simulink model "sensor_development"  (R2025b)
settings: Solver=VariableStepAuto  StartTime=0.0  StopTime=10.0  RelTol=1e-3
settings Model: Creator=atcushen  LastModifiedBy=atcushen

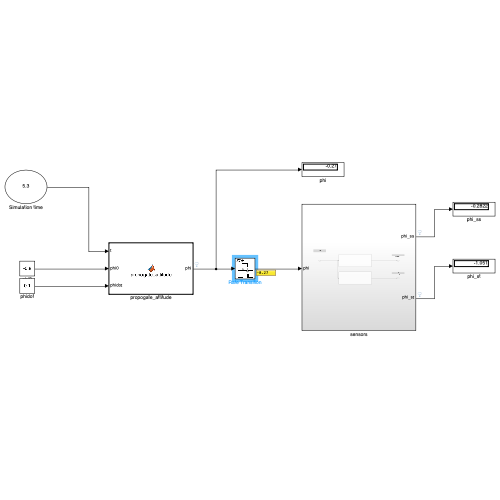
[thumbnail: Simulink's stored preview of the top-level diagram]
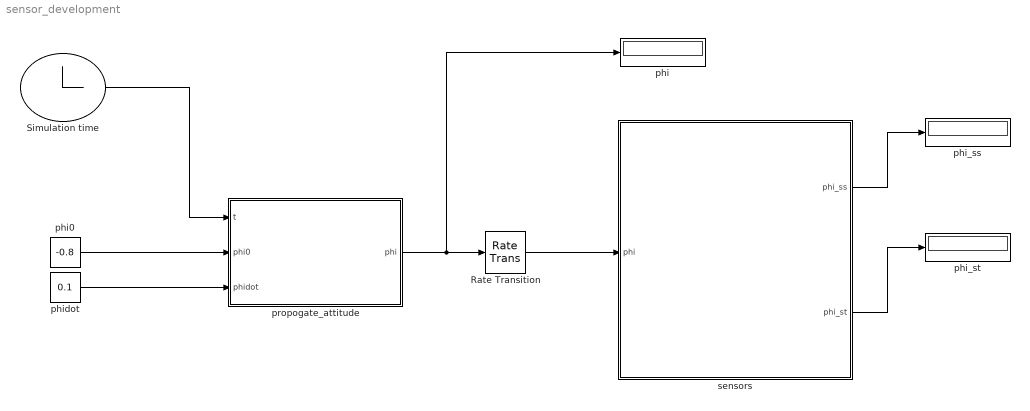
== system sensor_development ==
  Rate Transition : RateTransition  OutPortSampleTime=0.1
  Simulation time : Clock
  phi : Display
  phi0 : Constant  Value=-0.8
  phi_ss : Display
  phi_st : Display
  phidot : Constant  Value=0.1
  propogate_attitude : MATLAB Function  TreatAsAtomicUnit=on
  sensors : Subsystem
  wires:
  Simulation time/1 -> propogate_attitude/1(t)
  phi0/1 -> propogate_attitude/2(phi0)
  phidot/1 -> propogate_attitude/3(phidot)
  propogate_attitude/1(phi) -> phi/1, Rate Transition/1
  Rate Transition/1 -> sensors/1(phi)
  sensors/1(phi_ss) -> phi_ss/1
  sensors/2(phi_st) -> phi_st/1

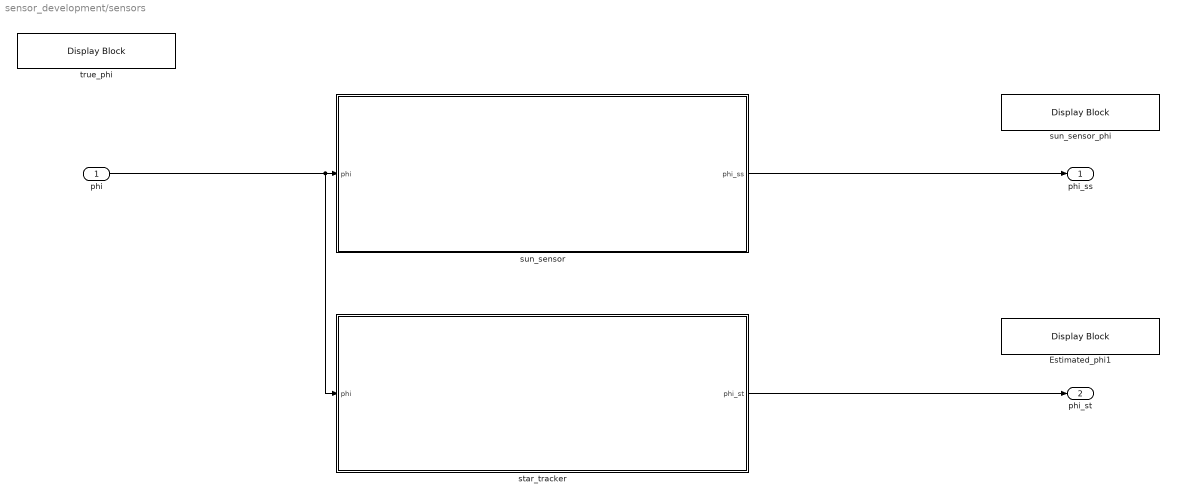
== system sensor_development/sensors ==
  phi : Inport
  Estimated_phi1 : DisplayBlock  LabelPosition=Bottom  Transparency=1  GridColor=[0.502, 0.502, 0.502]
  star_tracker : Subsystem
  sun_sensor : Subsystem
  sun_sensor_phi : DisplayBlock  LabelPosition=Bottom  Transparency=1  GridColor=[0.502, 0.502, 0.502]
  true_phi : DisplayBlock  LabelPosition=Hide  Transparency=1  GridColor=[0.502, 0.502, 0.502]
  phi_ss : Outport
  phi_st : Outport  Port=2
  wires:
  phi/1 -> star_tracker/1(phi), sun_sensor/1(phi)
  sun_sensor/1(phi_ss) -> phi_ss/1
  star_tracker/1(phi_st) -> phi_st/1

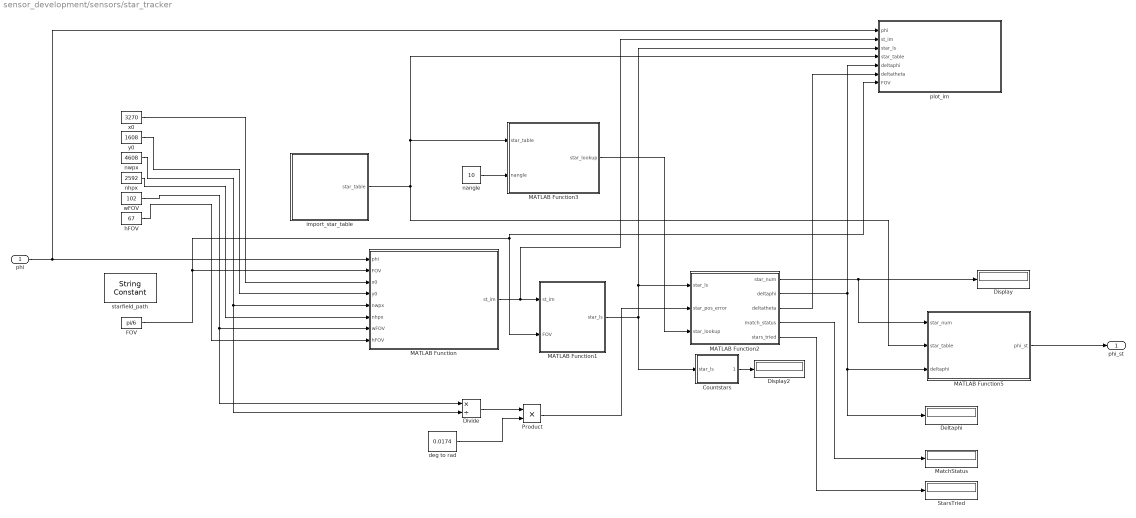
== system sensor_development/sensors/star_tracker ==
  phi : Inport
  Countstars : MATLAB Function  TreatAsAtomicUnit=on
  Deltaphi : Display
  Display : Display
  Display2 : Display
  Divide : Product  Inputs=*/
  FOV : Constant  Value=pi/6
  MATLAB Function : MATLAB Function  TreatAsAtomicUnit=on
  MATLAB Function1 : MATLAB Function  TreatAsAtomicUnit=on
  MATLAB Function2 : MATLAB Function  TreatAsAtomicUnit=on
  MATLAB Function3 : MATLAB Function  TreatAsAtomicUnit=on
  MATLAB Function5 : MATLAB Function  TreatAsAtomicUnit=on
  MatchStatus : Display
  Product : Product
  StarsTried : Display
  deg to rad : Constant  Value=0.0174
  hFOV : Constant  Value=67
  import_star_table : MATLAB Function  TreatAsAtomicUnit=on
  nangle : Constant  Value=10
  nhpx : Constant  Value=2592
  nwpx : Constant  Value=4608
  plot_im : MATLAB Function  TreatAsAtomicUnit=on
  starfield_path : StringConstant  String='star_field1.png'
  wFOV : Constant  Value=102
  x0 : Constant  Value=3270
  y0 : Constant  Value=1608
  phi_st : Outport
  wires:
  nhpx/1 -> MATLAB Function/6(nhpx)
  Countstars/1(num_stars) -> Display2/1
  nangle/1 -> MATLAB Function3/2(nangle)
  hFOV/1 -> MATLAB Function/8(hFOV)
  MATLAB Function2/4(match_status) -> MatchStatus/1
  Product/1 -> MATLAB Function2/2(star_pos_error)
  y0/1 -> MATLAB Function/4(y0)
  MATLAB Function1/1(star_ls) -> Countstars/1(star_ls), plot_im/3(star_ls), MATLAB Function2/1(star_ls)
  MATLAB Function/1(st_im) -> plot_im/2(st_im), MATLAB Function1/1(st_im)
  MATLAB Function3/1(star_lookup) -> MATLAB Function2/3(star_lookup)
  nwpx/1 -> Divide/2, MATLAB Function/5(nwpx)
  Divide/1 -> Product/1
  MATLAB Function2/5(stars_tried) -> StarsTried/1
  x0/1 -> MATLAB Function/3(x0)
  phi/1 -> plot_im/1(phi), MATLAB Function/1(phi)
  MATLAB Function2/2(deltaphi) -> Deltaphi/1, MATLAB Function5/3(deltaphi), plot_im/5(deltaphi)
  wFOV/1 -> Divide/1, MATLAB Function/7(wFOV)
  deg to rad/1 -> Product/2
  MATLAB Function2/1(star_num) -> MATLAB Function5/1(star_num), Display/1
  import_star_table/1(star_table) -> plot_im/4(star_table), MATLAB Function3/1(star_table), MATLAB Function5/2(star_table)
  FOV/1 -> MATLAB Function/2(FOV), MATLAB Function1/2(FOV), plot_im/7(FOV)
  MATLAB Function5/1(phi_st) -> phi_st/1
  MATLAB Function2/3(deltatheta) -> plot_im/6(deltatheta)

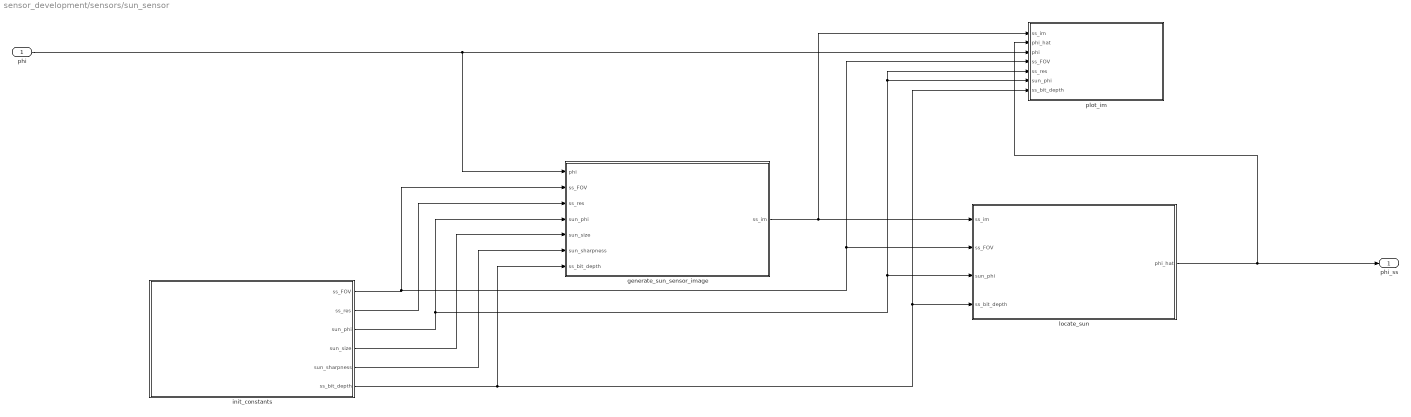
== system sensor_development/sensors/sun_sensor ==
  phi : Inport
  generate_sun_sensor_image : MATLAB Function  TreatAsAtomicUnit=on
  init_constants : MATLAB Function  TreatAsAtomicUnit=on
  locate_sun : MATLAB Function  TreatAsAtomicUnit=on
  plot_im : MATLAB Function  TreatAsAtomicUnit=on
  phi_ss : Outport
  wires:
  phi/1 -> generate_sun_sensor_image/1(phi), plot_im/3(phi)
  init_constants/5(sun_sharpness) -> generate_sun_sensor_image/6(sun_sharpness)
  generate_sun_sensor_image/1(ss_im) -> plot_im/1(ss_im), locate_sun/1(ss_im)
  locate_sun/1(phi_hat) -> phi_ss/1, plot_im/2(phi_hat)
  init_constants/1(ss_FOV) -> plot_im/4(ss_FOV), locate_sun/2(ss_FOV), generate_sun_sensor_image/2(ss_FOV)
  init_constants/2(ss_res) -> generate_sun_sensor_image/3(ss_res)
  init_constants/4(sun_size) -> generate_sun_sensor_image/5(sun_size)
  init_constants/3(sun_phi) -> generate_sun_sensor_image/4(sun_phi), plot_im/6(sun_phi), plot_im/5(ss_res), locate_sun/3(sun_phi)
  init_constants/6(ss_bit_depth) -> generate_sun_sensor_image/7(ss_bit_depth), plot_im/7(ss_bit_depth), locate_sun/4(ss_bit_depth)

== matlab function sensor_development/sensors/sun_sensor/plot_im ==
  data: ss_im input; phi_hat input; phi input; ss_FOV input; ss_res input; sun_phi input; ss_bit_depth input
function plot_im(ss_im,phi_hat,phi,ss_FOV,ss_res,sun_phi,ss_bit_depth)
   % Show synthetic image
    subplot(1, 2, 1);
    hold on
    imshow(ss_im, [], 'XData', linspace(-ss_FOV/2,ss_FOV/2,ss_res), 'YData', linspace(-ss_FOV/2,ss_FOV/2,ss_res));
    caxis([0 ss_bit_depth]); % Set the color axis limits for imshow
    % Add a vertical red line at (sun_phi - phi_hat)
    if ~isnan(phi_hat)
        xline(sun_phi - phi_hat, 'r', 'LineWidth', 2);
    end
    xline(sun_phi - phi, 'g', 'LineWidth', 2);
    set(gca, 'YDir', 'normal');
    title('Star Tracker Image'); % Title for the second subplot
    axis on
    xlabel('Azimuth (\delta\phi)');
    ylabel('Inclination (\delta\theta)');
    hold off
end

== matlab function sensor_development/sensors/star_tracker/MATLAB Function2 ==
  data: star_ls input; star_num output int32 size=1; star_pos_error input; star_lookup input; deltaphi output size=1; deltatheta output size=1; match_status output; stars_tried output
function [star_num,deltaphi,deltatheta,match_status,stars_tried] = match_to_lookup(star_ls,star_pos_error,star_lookup)
    % Input
    % star_ls: nx2 array, the phi and theta positions (relative to the
    % center of the image) for each star identified
    % star_pos_error: float, angular uncertainty in position of stars
    % star_lookup: nxnagle array, each row corresponds to given row in
    % star_table, columns are angular distances to closest stars

    % Output
    % star_num: integer, index number of matched star
    % deltaphi: float, offset in phi of matched star from image center, in
    % radians
    % deltatheta: float, offset in phi of matched star from image center,
    % in radians
    % CHANGED FOR CODEGEN - Initialize outputs with default values
    star_num = int32(-1);
    deltaphi = 0.0;
    deltatheta = 0.0;
    match_status = int32(0);  % debug output
    stars_tried = int32(0);   % debug output

    % Iterate through stars in image, starting closest to middle, until we
    % get a positive match
    star_match = false;
    
    % Calculate the sum of squares for each star position
    star_ls_dist = sum(star_ls.^2, 2);
    
    % Sort the star_ls based on the sum of squares
    [~, sorted_indices] = sort(star_ls_dist);
    star_ls = star_ls(sorted_indices, :);

    istar = 1;
    while star_match == false && istar <= length(star_ls)
        stars_tried = int32(istar);  % tracking progress
        
        % Compute distances to other stars
        phi_diff = star_ls(istar, 1) - star_ls(:, 1);
        theta_diff = star_ls(istar, 2) - star_ls(:, 2);
        angle_diff = sqrt(phi_diff.^2 + theta_diff.^2);

        % Sort the computed angular distances from smallest to largest
        [sorted_angles, ~] = sort(angle_diff);
        
        % Drop the first element of sorted_angles (distance to itself = 0)
        sorted_angles(1) = [];

        % Reduce sorted angles to only be as long as star_lookup is wide
        sorted_angles = sorted_angles(1:min(length(sorted_angles), size(star_lookup, 2)));

        % Create an array of stars within the positional error range
        match_indices = star_lookup(:, 1) >= (sorted_angles(1) - star_pos_error) & ...
                        star_lookup(:, 1) <= (sorted_angles(1) + star_pos_error);
        matched_stars = star_lookup(match_indices, :);

        % Check if that immediately identified the current state. 
        % If not, compare the angular distances one by one, bringing in more to
        % reduce the number of remaining options
        iangle = 2;

        while size(matched_stars,1) > 1 & iangle <= size(star_lookup,2)
            match_status = int32(2);  % indicates multiple matches being refined
            
            % We loop through the remaining matches
            for j = 1:size(match_indices, 1)
                if j ~= 0
                    % Check to see if the next closest star is within error of
                    % any of the neighbouring stars listed in the lookup table
                    % If none of the angles are close enough, then reject this
                    % match
                    if all(abs(star_lookup(j, iangle:end) - sorted_angles(iangle)) > star_pos_error)
                        match_indices(j) = 0; % Set the jth non-zero element of match_indices to zero
                    end
                end 
            end
            matched_stars = star_lookup(match_indices, :);
        
            iangle = iangle + 1;
        end
        
        % Check if we could use this star 
        if size(matched_stars,1) ~= 1
            % no match found for this star, continue
            istar = istar + 1; % Move to the next star
        else
            % CHANGED FOR CODEGEN - Force scalar by using loop instead of find
            for k = 1:length(match_indices)
                if match_indices(k) ~= 0
                    star_num = int32(k);
                    break;
                end
            end
            deltaphi = star_ls(istar,1); % Offset in phi
            deltatheta = star_ls(istar,2); % Offset in theta
            star_match = true;
            match_status = int32(1);  % successful match
        end
    end
    
    % Return error if star tracker failed 
    if star_match == false
        % CHANGED FOR CODEGEN - tracker failed
        star_num = int32(-1);
        deltaphi = 0.0;
        deltatheta = 0.0;
        match_status = int32(0);  % Failed to match
    end
    
end

== matlab function sensor_development/sensors/star_tracker/MATLAB Function5 ==
  data: star_num input; phi_st output; star_table input; deltaphi input
function phi_st = compute_boresight_phi(star_num,star_table,deltaphi)
    % Input
    % star_num: integer, index number of matched star
    % star_table: n_stars x 3 array, where column 1 is phi position of
    % star, column 2 is theta position, column 3 is relative brightness
    % deltaphi: float, offset in phi of matched star from image center, in
    % radians
    
    % Output
    % boresight_phi: float, actual orientation of the center of the cameras
    % FOV [rad]
    
    if star_num<0
        phi_st = NaN;
    else
        phi_st = star_table(star_num,1) - deltaphi;
    end
end

== matlab function sensor_development/sensors/star_tracker/Countstars ==
  data: star_ls input; num_stars output
function num_stars = count_stars(star_ls)
    num_stars = int32(size(star_ls, 1));
end

== matlab function sensor_development/sensors/star_tracker/import_star_table ==
  data: star_table output size=73,2 [..200]
function star_table = import_star_table()
    % Output:
    % star_table: n_stars x 2 array, where column 1 is phi position of
    % star, column 2 is theta position, in radians

    struct = load("star_table2.mat");
    star_table = struct.star_table;
    
end

== matlab function sensor_development/sensors/star_tracker/MATLAB Function ==
  data: st_im output; phi input; FOV input; x0 input; y0 input; nwpx input; nhpx input; wFOV input; hFOV input
function st_im  = crop_starfield(phi,FOV,x0,y0,nwpx,nhpx,wFOV,hFOV)
    % Input
    % image: str, path to .png field to import of starfield
    % phi: float, boresight angle of camera, in radians, from -pi to pis
    % FOV: float, angular field of view of camera, in radians, from 0 to 2pi
    % x0: int, x pixel coord of reference star 
    % y0: int, x pixel coord of reference star 
    % nwpx: int, number of pixels of width of starfield image
    % nhpx: int, number of pixels of height of starfield image
    % wFOV: float, field of view width of starfield image [deg]
    % hFOV: float, field of view height of starfield image [deg]
    % Output:
    % st_im: nres x nres array, representing synethic star tracker image

    %starfield_path = '/Users/atcushen/Documents/MATLAB/scripts/star_field1.mat';
    starfield_path = 'star_field2.mat';

    % Load the .png image as a black and white image array
    %img = imread(starfield_path); % Read the image from the specified path
    file = load(starfield_path);
    img = file.img; 
    starfield_im = rgb2gray(img); % Convert the image to grayscale
    starfield_im = flip(starfield_im,1); % Image array is upside down)

    % Create coordinate axes
    x_ax = linspace(1,nwpx,nwpx) - x0;
    y_ax = linspace(1,nhpx,nhpx) - y0;
    phi_ax = x_ax * pi/180 * wFOV/nwpx;
    theta_ax = y_ax * pi/180 * hFOV/nhpx;
    
    % Crop the starfield image based on the field of view and the phi axis
    phi_indices = phi_ax >= (phi - FOV/2) & phi_ax <= (phi + FOV/2);
    theta_indices = theta_ax >= (-FOV/2) & theta_ax <= (FOV/2); %y0-round(nres/2):y0-round(nres/2)+nres-1;
    
    % Ensure indices are within bounds
    %phi_indices = max(min(phi_indices, nwpx), 1);
    %theta_indices = max(min(theta_indices, nhpx), 1);
    
    % Crop the image
    st_im = starfield_im(theta_indices, phi_indices);
end

== matlab function sensor_development/sensors/star_tracker/MATLAB Function1 ==
  settings: updateMethod=DISCRETE  sampleTime=0.1
  data: st_im input; star_ls output size=[200 2]; FOV input
function star_ls = identify_stars(st_im, FOV)
 % Input:
% st_im: nxn array, representing image from star tracker
% FOV: float, field of view along each edge of image
% Output:
% star_ls: nx2 array, the phi and theta positions (relative to the
% center of the image) for each star identified

% Get image dimensions (not passed to function call)
[theta_nres,phi_nres] = size(st_im);

% Convert coordinates to phi and theta positions
phi_positions = linspace(-FOV/2, FOV/2, phi_nres);
theta_positions = linspace(-FOV/2, FOV/2, theta_nres);

% Identify bright points in the star tracker image
 threshold = 0.3 * 255; % Set a threshold to identify bright points
% Create filtered im
 filtered_im = zeros(size(st_im)); % Initialize filtered image
 filtered_im(st_im > threshold) = 1; % Set values to 1 where st_im exceeds threshold
% Find connected components
 CC = bwconncomp(filtered_im);
% Create label matrix - CHANGED FOR CODEGEN
 L = zeros(size(filtered_im), 'uint16');
 for k = 1:CC.NumObjects
     L(CC.PixelIdxList{k}) = k;
 end
% Create output array for star positions
 star_ls = zeros(max(L(:)), 2);
% Iterate through each connected component
for istar = 1:max(L(:))
% Get the coordinates of the current star cluster
 [y_cluster, x_cluster] = find(L == istar);
% Store the average position of the cluster
 star_ls(istar, 1) = mean(phi_positions(x_cluster)); % Average phi coordinate
 star_ls(istar, 2) = mean(theta_positions(y_cluster)); % Average theta coordinate
end
end

== matlab function sensor_development/propogate_attitude ==
  data: t input; phi output; phi0 input; phidot input
% propogate attitude
function phi = propogate_attitude(t,phi0,phidot)
    % Input: 
    % t: float, current time, in s
    % phi0: float, initial attitude, in radians
    % phidot: float, rotation rate, in rad/sec
    
    % Output:
    % phi: float, current attitude, in rad/sec

    phi = mod(t*phidot + phi0 + pi,2*pi) - pi;
end

== matlab function sensor_development/sensors/star_tracker/plot_im ==
  data: phi input; st_im input; star_ls input; star_table input; deltaphi input; deltatheta input; FOV input
function plot_im(phi,st_im,star_ls,star_table,deltaphi,deltatheta,FOV)
    [theta_nres,phi_nres] = size(st_im);
   % Create a subplot for the synthetic star tracker image
    subplot(1, 2, 2);
    hold on
    imshow(st_im, [], 'XData', linspace(-FOV/2,FOV/2,phi_nres), 'YData', linspace(-FOV/2,FOV/2,theta_nres));
    caxis([0 255])
    set(gca, 'YDir', 'normal');
    scatter(star_ls(:, 1), star_ls(:, 2), 200, 'yellow', 'MarkerEdgeColor', 'yellow', 'MarkerFaceColor', 'none');
    scatter(deltaphi, deltatheta, 200, 'green', 'MarkerEdgeColor', 'green', 'MarkerFaceColor', 'none');
    scatter(star_table(:,1)-phi, star_table(:,2), 250, 'red', 'MarkerEdgeColor', 'red', 'MarkerFaceColor', 'none');
    scatter(deltaphi, deltatheta, 200, 'green', 'MarkerEdgeColor', 'green', 'MarkerFaceColor', 'none', 'Marker', 'x');
    hold off
    title('Star Tracker Image'); % Title for the second subplot
    axis on
    xlim([-FOV/2, FOV/2]); % Set x-axis limits from -FOV/2 to FOV/2
    xlabel('Azimuth (\delta\phi)');
    ylabel('Inclination (\delta\theta)');

end

== matlab function sensor_development/sensors/star_tracker/MATLAB Function3 ==
  data: star_table input; star_lookup output; nangle input
function star_lookup = generate_star_lookup_table(star_table, nangle)
    % Input
    % star_table: nx3 array, from generate_star_table
    % nangle: integer, how many stars to compute angles to from reference
    % star

    % Output
    % star_lookup: nxnagle array, each row corresponds to given row in
    % star_table, columns are angular distances to nangle closest stars

    % Initialize lookup table
    star_lookup = zeros(size(star_table, 1), nangle);

    % Iterate through each star in the table
    for istar = 1:length(star_table)
        
        % Compute the angular distances from the current star to all other stars
        phi_diff = star_table(istar, 1) - star_table(:, 1);
        theta_diff = star_table(istar, 2) - star_table(:, 2);
        angle_diff = sqrt(phi_diff.^2 + theta_diff.^2);

        % Sort the angular distances and get the indices of the smallest values
        [sorted_angles, ~] = sort(angle_diff);
        star_lookup(istar, :) = sorted_angles(2:min(nangle+1, length(sorted_angles))); % Store the smallest values
    end
end

== matlab function sensor_development/sensors/sun_sensor/generate_sun_sensor_image ==
  data: phi input; ss_im output size=64,64; ss_FOV input; ss_res input; sun_phi input; sun_size input; sun_sharpness input; ss_bit_depth input
% Generate a synthetic sun sensor IR image, based off present attitude phi
function ss_im = generate_sun_sensor_image(phi,ss_FOV,ss_res,sun_phi,sun_size,sun_sharpness,ss_bit_depth)
    % Input: 
    % phi: float, current pointing angle, in radians
    % ss_FOV: float, viewing angle of sun sensor in radians
    % ss_res: integer, number of pixels on edge of image
    % sun_phi: float, angular position of sun in radians
    % sun_size: float, angular size of sun in radians
    % sun_sharpness: float, degree of function describing sun shape (higher
    % is sharper), recommended 1-5
    % ss_bit_depth: integer, max brightness value of each pixel
    
    % Output:
    % ss_im: ss_res x ss_res array representing synthetic sun sensor image

    phi_ax = linspace(phi-ss_FOV/2,phi+ss_FOV/2,ss_res); % Determine phi axis of image
    theta_ax = linspace(-ss_FOV/2,ss_FOV/2,ss_res); % Determine theta axis of image

    [phi_im, theta_im] = meshgrid(phi_ax, theta_ax); % Create 2D array of angle coordinates
    
    % Add the sun to the image
    ss_im = ss_bit_depth * exp(-((((phi_im-sun_phi).^2+theta_im.^2)/sun_size^2).^sun_sharpness));

    % Add random noise to the image 
    noise_level = ss_bit_depth*0.05; % Adjust the noise level as needed
    noise = noise_level * randn([ss_res,ss_res]); % Generate Gaussian noise
    ss_im = ss_im + noise; % Add noise to the image
    ss_im(ss_im < 0) = 0; % Ensure no negative value
end

== matlab function sensor_development/sensors/sun_sensor/init_constants ==
  data: ss_FOV output; ss_res output; sun_phi output; sun_size output; sun_sharpness output; ss_bit_depth output
% define all our constants
function [ss_FOV,ss_res,sun_phi,sun_size,sun_sharpness,ss_bit_depth] = init_constants
    % Output
    ss_FOV = pi/4;  % float, sun sensor field of field, in radians 
    ss_res = 64; % int, number of pixels on a side of sun sensor image
    sun_phi = 0; % float, position of sun in sky, in radians
    sun_size = pi/128; % float, angular size of sun, in radians
    sun_sharpness = 3; % float, sun sharpness factor (1-5)
    ss_bit_depth = 63; % int, maximum pixel value of sun sensor image
end

== matlab function sensor_development/sensors/sun_sensor/locate_sun ==
  data: ss_im input; phi_hat output; ss_FOV input; sun_phi input; ss_bit_depth input
function phi_hat = locate_sun(ss_im,ss_FOV,sun_phi,ss_bit_depth) 
    % Input: 
    % ss_im: ss_res x ss_res array representing synthetic sun sensor image
    % ss_FOV: float, viewing angle of sun sensor in radians (assumed
    % square)
    % sun_phi: float, absolute angular position of sun in sky, in radians
    % ss_bit_depth: integer, max brightness value of each pixel
    
    % Output: 
    % phi_hat: float, estimate for current attitude, in radians
    
    % Set threshold; cells dimmer than this will be assumed to not be the
    % sun
    cutoff_brightness = 0.05 * ss_bit_depth;
    
    % Get dimensions of the image
    [~,ss_res] = size(ss_im);
    
    % Sum ss_im along columns to get the total pixel brightness in each column
    col_brightness = sum(ss_im, 1); % Sum along rows to get a 1D array

    % Filter out false negatives
    col_brightness(col_brightness < ss_res * cutoff_brightness) = 0;
     
    % Check for adjacent entries in col_brightness greater than zero
    adjacent_found = false;
    multiple_adjacents = false;
    for i = 1:length(col_brightness)-1
        if col_brightness(i) > 0 && col_brightness(i+1) > 0
            if adjacent_found && col_brightness(i-1) == 0
                multiple_adjacents = true;
            else
                adjacent_found = true;
            end
        end
    end
    
    % Display errors
    if ~adjacent_found 
        disp('ERROR: No sun found in frame');
        phi_hat = NaN; % Return NaN if no adjacent entries are found
        return; % Exit the function early
    elseif multiple_adjacents
        disp('ERROR: Multiple sun-like clusters found, cannot identify the sun');
        phi_hat = NaN; % Return NaN if multiple adjacent entries are found
        return; % Exit the function early
    end
    
    % Iterate over the indices of col_brightness that are greater than zero
    sun_indices = find(col_brightness > 0);
       
    % Get the brightness-weighted pixel location of the sun
    sun_pixel_loc = sum(col_brightness(sun_indices) .* sun_indices) / sum(col_brightness(sun_indices));

    % Determine phi_hat from this relative position
    phi_hat = sun_phi - ((sun_pixel_loc / ss_res) * ss_FOV - ss_FOV/2); % Estimate current attitude
   
end
